simulink model "TST_ACT_MAG"  (Simulink 9.0)
settings: Solver=VariableStepAuto  StartTime=0.0  StopTime=10000  RelTol=1e-3
libraries: ACT_MAG x1, DYN_MAG x1, DYN_TIME x1
settings Model: Creator=Mahal  LastModifiedBy=Mahal
settings DataIOCC: SaveFormat=Dataset
settings OptimizationCC: LifeSpan=auto
settings DebuggingCC: UnderspecifiedInitializationDetection=Simplified  MergeDetectMultiDrivingBlocksExec=error  SFUnexpectedBacktrackingDiag=error  SFNoUnconditionalDefaultTransitionDiag=error  SFExecutionAtInitializationDiag=warning
settings HardwareCC: ProdBitPerPointer=64  ProdBitPerSizeT=64  ProdBitPerPtrDiffT=64  ProdLargestAtomicFloat=Float  ProdIntDivRoundTo=Zero  ProdEndianess=LittleEndian  ProdWordSize=64  ProdHWDeviceType=Intel->x86-64 (Windows64)
settings ModelReferenceCC: PropagateSignalLabelsOutOfModel=on
settings CodeAppCC: StateflowObjectComments=off
settings GRTTargetCC: TargetLangStandard=C99 (ISO)
settings ConfigComp: CovMetricSettings=dwe  CovHtmlReporting=off  CovSaveCumulativeToWorkspaceVar=off  CovSaveSingleToWorkspaceVar=off  CovExternalEMLEnable=on

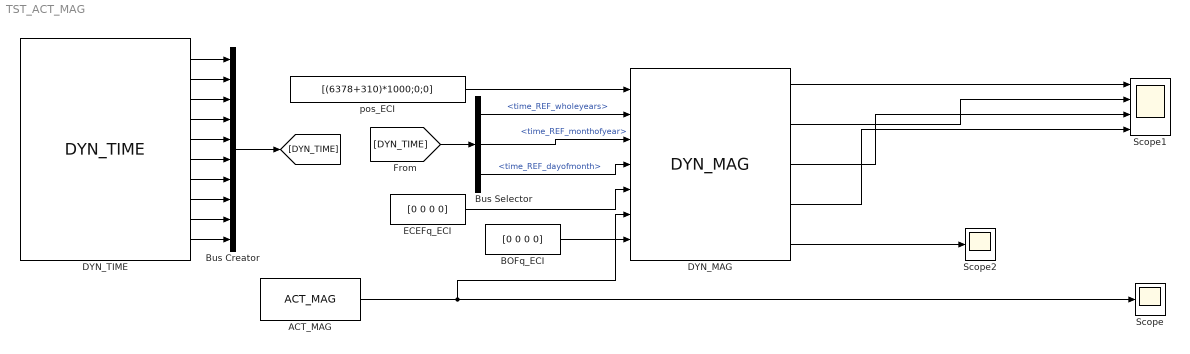
== system TST_ACT_MAG ==
  ACT_MAG : ACT_MAG/ACT_MAG
  BOFq_ECI : Constant  Value=[0 0 0 0]
  Bus Creator : BusCreator  Inputs=10
  Bus Selector : BusSelector  OutputSignals=time_REF_wholeyears,time_REF_monthofyear,time_REF_dayofmonth
  DYN_MAG : DYN_MAG/DYN_MAG
  DYN_TIME : DYN_TIME/DYN_TIME
  ECEFq_ECI : Constant  Value=[0 0 0 0]
  Scope : Scope
  Scope1 : Scope  NumInputPorts=4
  Scope2 : Scope
  pos_ECI : Constant  Value=[(6378+310)*1000;0;0]
  wires:
  DYN_MAG/4 -> Scope1/4
  Bus Creator/1 -> [DYN_TIME]
  ECEFq_ECI/1 -> DYN_MAG/5
  DYN_TIME/10 -> Bus Creator/10
  DYN_TIME/1 -> Bus Creator/1
  Bus Selector/2 -> DYN_MAG/3  "<time_REF_monthofyear>"
  DYN_TIME/4 -> Bus Creator/4
  DYN_TIME/5 -> Bus Creator/5
  Bus Selector/3 -> DYN_MAG/4  "<time_REF_dayofmonth>"
  Bus Selector/1 -> DYN_MAG/2  "<time_REF_wholeyears>"
  DYN_MAG/2 -> Scope1/2
  DYN_TIME/9 -> Bus Creator/9
  [DYN_TIME] -> Bus Selector/1
  DYN_TIME/3 -> Bus Creator/3
  BOFq_ECI/1 -> DYN_MAG/6
  DYN_TIME/8 -> Bus Creator/8
  DYN_TIME/6 -> Bus Creator/6
  DYN_MAG/1 -> Scope1/1
  pos_ECI/1 -> DYN_MAG/1
  DYN_TIME/7 -> Bus Creator/7
  DYN_TIME/2 -> Bus Creator/2
  DYN_MAG/3 -> Scope1/3
  ACT_MAG/1 -> DYN_MAG/7, Scope/1
  DYN_MAG/5 -> Scope2/1
